simulink library "commchan2"  (Simulink 6.0)
settings: Solver=ode45  SolverMode=SingleTasking  StartTime=0.0  StopTime=10.0  RelTol=1e-3
undefined symbols (not defined in the file or in its folder): j, params
libraries: dspmlti3 x5, dspsigattribs x4, dspsrcs4 x3, commblksprivate x2, dspmtrx3 x2, dsparch4 x1, dspsigops x1, commchan2 x1
settings Model: RequirementInfo=9  CovMetricSettings=d  Creator=tdelve  LastModifiedBy=cvora  ExtModeAutoUpdateStatusClock=off  ProdHWDeviceType=Specified
settings DataIOCC: SignalLoggingName=logsOut
settings OptimizationCC: BooleanDataType=off
settings DebuggingCC: CheckExecutionContextPreStartOutputMsg=on  CheckExecutionContextRuntimeOutputMsg=on  SolverPrmCheckMsg=none
settings HardwareCC: ProdHWDeviceType=Specified
settings SFSimCC: SFSimApplyToAllLibs=on  SFSimBuildMode=Incremental

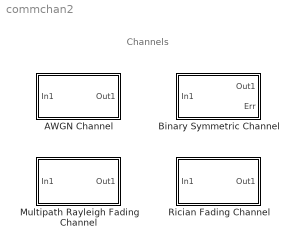
== system commchan2 ==
  note: Channels
  AWGN Channel : Subsystem  PropExecContextAcrossSSBoundary=on  mask(AWGN Channel){seed=67, noiseMode=Signal to noise ratio  (Eb/No), EbNodB=10, EsNodB=10, SNRdB=10, bitsPerSym=1, Ps=1, Tsym=1, variance=1}
      mask prompts: seed "Initial seed:"; noiseMode "Mode:"; EbNodB "Eb/No (dB):"; EsNodB "Es/No (dB):"; SNRdB "SNR (dB):"; bitsPerSym "Number of bits per symbol:"; Ps "Input signal power (watts):"; Tsym "Symbol period (s):"
      mask help:
      | Add white Gaussian noise to the input signal. The input and output signals can be real or complex. This block supports multichannel input and output signals as well as frame-based processing.
      |
      | When using either of the variance modes with complex inputs, the variance values are equally divided among the real and imaginary components of the input signal.
      mask init:
      | [mode,s]=commblkawgnchan2(gcb,'init');
      | if ~isempty(s.status) error(s.status); end
      mask Help: helpview(commbhelp)
      mask StyleString: edit,popup(Signal to noise ratio  (Eb/No)|Signal to noise ratio  (Es/No)|Signal to noise ratio  (SNR)|Variance from mask|Variance from port),edit,edit,edit,edit,edit,edit,edit
      mask CallbackString: |commblkawgnchan2(gcb,'Mode');|||||||
      mask Display:
      | plot(-10,-10,110, 110,[05 15 10 10 05 10 18 14 13 7.5 13 41 44 47 50 53 57
      | 59 100-[13 7.5 13 14 18 10 5 10 10 15 5]],[70 70 70 85 92 85 79 82 90 88.5
      | 90 90 87 93 87 93 87 90 90 88.5 90 82 79 85 92 85 70 70 70]);
      | disp('AWGN');
      | port_label('input',s.i1,s.i1s);
      | port_label('input',s.i2,s.i2s);
      | port_label('output',s.o1,s.o1s);
  Binary Symmetric Channel : Subsystem  PropExecContextAcrossSSBoundary=on  mask(Binary Symmetric Channel){P=0.05, s=71, E=on}
      mask prompts: P "Error probability:"; s "Initial seed:"; E "Output error vector"
      mask help:
      | Add binary errors to the input signal. The error probability can be a scalar or a vector with the same length as the input vector length.
      |
      | The optional second output is the error vector.
      mask init:
      | blk_icon = commblkbschan(P,s);
      mask Help: helpview(commbhelp)
      mask Display:
      | plot(0,0,100,100,[05 15 10 10 05 10 18 14 13 7.5 13 41 44 47 50 53 57 59 100-[13 7.5 13 14 18 10 5 10 10 15 5]],[70 70 70 85 92 85 79 82 90 88.5 90 90 87 93 87 93 87 90 90 88.5 90 82 79 85 92 85 70 70 70]);
      | disp('BSC')
      | port_label('output',blk_icon.portnum,blk_icon.portlabel);
  Multipath Rayleigh Fading Channel : Subsystem  PropExecContextAcrossSSBoundary=on  mask(Multipath Rayleigh Fading Channel){Fd=40, simTs=1e-6, delayVec=[0 2e-6], gainVecdB=[0 -3], normGain=on, Seed=73}
      mask prompts: Fd "Maximum Doppler shift (Hz):"; simTs "Sample time:"; delayVec "Delay vector (s):"; gainVecdB "Gain vector (dB):"; normGain "Normalize gain vector to 0 dB overall gain"; Seed "Initial seed:"
      mask help:
      | Multipath Rayleigh fading channel for complex baseband signals.
      |
      | Multiplies the input signal with samples of a Rayleigh distributed complex random process. The spectrum of the Rayleigh process is given by the Jakes PSD.
      |
      | The number of paths equals the length of either the 'Delay vector' or 'Gain vector' parameters.
      mask init:
      | commblkrayleighchan2(gcb);
      mask Help: helpview(commbhelp)
      mask Display:
      | plot(0,0,100,100,[05 15 10 10 05 10 18 14 13 7.5 13 41 44 47 50 53 57 59 100-[13 7.5 13 14 18 10 5 10 10 15 5]],[70 70 70 85 92 85 79 82 90 88.5 90 90 87 93 87 93 87 90 90 88.5 90 82 79 85 92 85 70 70 70]);
      | disp('Multipath\nRayleigh Fading')
  Rician Fading Channel : Subsystem  PropExecContextAcrossSSBoundary=on  mask(Rician Fading Channel){K=1, Fd=40, simTs=1e-6, delayVec=0, gainVecdB=0, Seed=79}
      mask prompts: K "K-factor:"; Fd "Maximum Doppler shift (Hz):"; simTs "Sample time:"; delayVec "Delay (s):"; gainVecdB "Gain (dB):"; Seed "Initial seed:"
      mask help:
      | Rician fading channel for complex baseband signals.
      |
      | Multiplies the input signal with samples of a Rician distributed complex random process. The K-factor parameter specifies the linear ratio of power in the direct path to the diffuse power.  The spectrum of the Rician process is given by the Jakes PSD.
      mask init:
      | commblkricianchan2(gcb);
      mask Help: helpview(commbhelp)
      mask Display:
      | plot(0,0,100,100,[05 15 10 10 05 10 18 14 13 7.5 13 41 44 47 50 53 57 59 100-[13 7.5 13 14 18 10 5 10 10 15 5]],[70 70 70 85 92 85 79 82 90 88.5 90 90 87 93 87 93 87 90 90 88.5 90 82 79 85 92 85 70 70 70]);
      | disp('Rician\nFading')

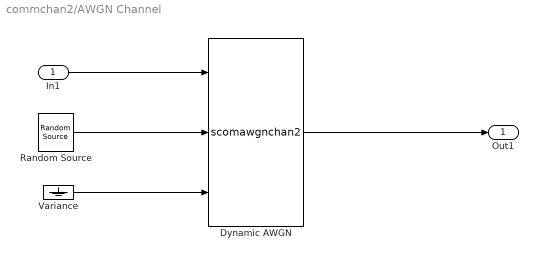
== system commchan2/AWGN Channel ==
  In1 : Inport  LatchInput=off
  Dynamic AWGN : S-Function  FunctionName=scomawgnchan2  Parameters=noiseMode, EbNodB, EsNodB, SNRdB, bitsPerSym, Ps, Tsym, variance
  Random Source : dspsrcs4/Random Source  SrcType=Gaussian  NormMethod=Ziggurat  CltLength=12  Min=0  Max=1  Mean=0  Var=1  RepMode=Specify seed  Seed=seed  Inherit=on  SampMode=Discrete  SampTime=1  SampFrame=1  DataType=Double  OutComplex=Real
  Variance : Ground
  Out1 : Outport
  wires:
  Random Source/1 -> Dynamic AWGN/2
  In1/1 -> Dynamic AWGN/1
  Dynamic AWGN/1 -> Out1/1
  Variance/1 -> Dynamic AWGN/3

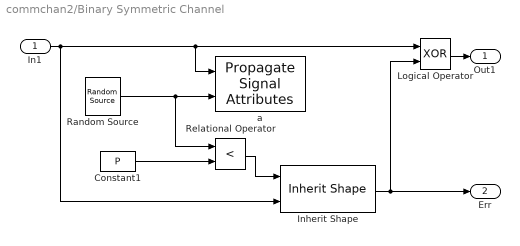
== system commchan2/Binary Symmetric Channel ==
  In1 : Inport  LatchInput=off
  Constant1 : Constant  Value=P
  Inherit Shape : commblksprivate/Inherit Shape
  Logical Operator : Logic  Operator=XOR  OutDataTypeMode=Specify via dialog  LogicDataType=float('double')
  Random Source : dspsrcs4/Random Source  SrcType=Uniform  NormMethod=Ziggurat  CltLength=12  Min=0  Max=1  Mean=0  Var=1  RepMode=Specify seed  Seed=s  Inherit=on  SampMode=Discrete  SampTime=1  SampFrame=1  DataType=Double  OutComplex=Real
  Relational Operator : RelationalOperator  Operator=<  LogicOutDataTypeMode=Specify via dialog  LogicDataType=float('double')  InputSameDT=on
  a : commblksprivate/Propagate Signal Attributes
  Out1 : Outport
  Err : Outport  Port=2
  wires:
  Relational Operator/1 -> Inherit Shape/1
  Inherit Shape/1 -> Logical Operator/2, Err/1
  Logical Operator/1 -> Out1/1
  In1/1 -> Inherit Shape/2, Logical Operator/1, a/1
  Constant1/1 -> Relational Operator/2
  Random Source/1 -> Relational Operator/1, a/2

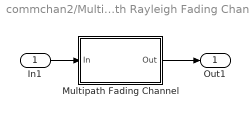
== system commchan2/Multipath Rayleigh Fading Channel ==
  In1 : Inport  LatchInput=off
  Multipath Fading Channel : Subsystem  PropExecContextAcrossSSBoundary=on  mask(Multipath Fading Channel){Fd=Fd, LOSFd=0, K=0, simTs=simTs, delayVec=delayVec, gainVecdB=gainVecdB, normGain=on, Seed=Seed}
      mask prompts: Fd "Doppler frequency (Hz):"; LOSFd "Line-of-sight Doppler frequency (Hz):"; K "K-factor:"; simTs "Sample time (sec):"; delayVec "Delay vector (sec):"; gainVecdB "Gain vector (dB):"; normGain "Normalize gain vector to 0 dB overall gain"; Seed "Initial seed:"
      mask help:
      | Multipath fading channel for complex baseband signals.
      |
      | Multiplies the input signal with samples of a complex random process. The spectrum of the random process is given by the Jakes PSD, where the Doppler frequency parameter determines the maximum Doppler frequency. The K-factor parameter specifies the linear ratio of power in the direct path to the diffuse power.
      |
      | The number of paths equals the length of either the 'Delay vector' or 'Gain vector' parameters.
      mask init:
      | [ecode,emsg,params] = commblkfadingchan2(gcb,Fd,LOSFd,K,simTs,delayVec,gainVecdB,normGain,Seed);
      | if(ecode==1)
      |     error(emsg);
      | elseif(ecode==2)
      |     warning(emsg);
      | end;
      mask Display:
      | plot(0,0,100,100,[05 15 10 10 05 10 18 14 13 7.5 13 41 44 47 50 53 57 59 100-[13 7.5 13 14 18 10 5 10 10 15 5]],[70 70 70 85 92 85 79 82 90 88.5 90 90 87 93 87 93 87 90 90 88.5 90 82 79 85 92 85 70 70 70]);
      | disp('Multipath\nFading')
  Out1 : Outport
  wires:
  In1/1 -> Multipath Fading Channel/1(In)
  Multipath Fading Channel/1(Out) -> Out1/1

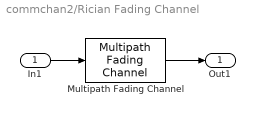
== system commchan2/Rician Fading Channel ==
  In1 : Inport  LatchInput=off
  Multipath Fading Channel : commchan2/Multipath Rayleigh Fading Channel/Multipath Fading Channel  Fd=Fd  LOSFd=0  K=K  simTs=simTs  delayVec=delayVec  gainVecdB=gainVecdB  normGain=off  Seed=Seed
  Out1 : Outport
  wires:
  In1/1 -> Multipath Fading Channel/1
  Multipath Fading Channel/1 -> Out1/1

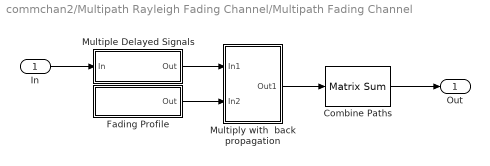
== system commchan2/Multipath Rayleigh Fading Channel/Multipath Fading Channel ==
  In : Inport  LatchInput=off
  Combine Paths : dspmtrx3/Matrix Sum  DialogController=dspDDGCreate  DialogControllerArgs=DataTag0  Dim=Rows  roundingMode=Floor  overflowMode=off
  Fading Profile : Subsystem  PropExecContextAcrossSSBoundary=on
      mask Display: disp('Fading\nProfile')
  Multiple Delayed Signals : Subsystem  PropExecContextAcrossSSBoundary=on  mask(Multiple Delayed Signals){delayVector=params.sampleDelayVec, Ts=simTs}
      mask prompts: delayVector "Path delay vector:"; Ts "Sample time (sec):"
      mask init:
      | nPaths = length(delayVector);
      | maxDelay = ceil(max(delayVector))+1;
      mask Display: disp('Multiple\ndelayed signals');
  Multiply with  back propagation : Subsystem  PropExecContextAcrossSSBoundary=on  mask(Multiply with back propagation){propTarget=Input 2, Ts=simTs, numChan=params.nPaths}
      mask prompts: propTarget "Propagation target:"; Ts "Sample time:"; numChan "Number of channels:"
      mask help:
      | Perform multiplication of the two input signals.
      |
      | The width and complexity of the output and the port not targeted for propagation must be identical. The width and complexity of the port targeted for propagation is set to that of the other input.
      |
      | The block sample time is the product of the number of samples per frame and the sample time parameter.
      mask StyleString: popup(Input 1|Input 2),edit,edit
      mask Display: disp('Multiply\nwith prop');
  Out : Outport
  wires:
  Multiple Delayed Signals/1(Out) -> Multiply with  back propagation/1(In1)
  Fading Profile/1(Out) -> Multiply with  back propagation/2(In2)
  In/1 -> Multiple Delayed Signals/1(In)
  Multiply with  back propagation/1(Out1) -> Combine Paths/1
  Combine Paths/1 -> Out/1

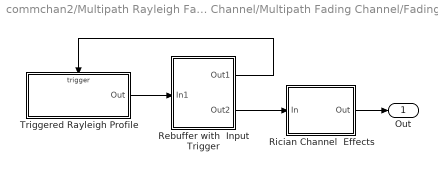
== system commchan2/Multipath Rayleigh Fading Channel/Multipath Fading Channel/Fading Profile ==
  Rebuffer with  Input Trigger : Subsystem  PropExecContextAcrossSSBoundary=on  mask(Rebuffer with Input Trigger){startSample=params.startDelay, numChan=params.nPaths, inputWidthMode=Based on output width, inputWidth=params.intFactor, inputWidthMin=params.intFactor, inputWidthStep=params.intFactor}
      mask prompts: startSample "Start delay:"; numChan "Number of channels:"; inputWidthMode "Input width mode:"; inputWidth "Input width (per channel):"; inputWidthMin "Minimum input width (per channel):"; inputWidthStep "Input width step size (per channel):"
      mask help: This block inherits the input and output port widths and complexity and the output sample time. The input must be from a function call subsystem. The block generates a function call trigger on port 1 when ever data is required. and outputs the buffered input data on port 2.
      mask init:
      | s = commblktriggeredbuffer(gcb,'init',{});
      mask StyleString: edit,edit,popup(Inherit|Specify|Based on output width),edit,edit,edit
      mask CallbackString: ||commblktriggeredbuffer(gcb,'InputWidthMode');|||
      mask Display:
      | disp('Rebuffer\nwith trigger');
      | port_label('input',s.i1,s.i1s);
      | port_label('output',s.o1,s.o1s);
      | port_label('output',s.o2,s.o2s);
  Rician Channel  Effects : Subsystem  PropExecContextAcrossSSBoundary=on  mask(Ricean Channel Effects){Doppler=params.LOSFd, K=params.K, opPower=params.gainVecLin, Ts=simTs, numChan=params.nPaths}
      mask prompts: Doppler "Line-of-sight Doppler frequency (Hz):"; K "K-factor"; opPower "Required output power (Watts):"; Ts "Sample time (s):"; numChan "Number of channels:"
      mask help: Add a complex phasor to the unity variance complex input to produce Rician channel effects. The Doppler frequency parameter determines frequency of the complex phasor.
      mask Display: disp('Rician\nChannel')
  Triggered Rayleigh Profile : Subsystem  TreatAsAtomicUnit=on  PropExecContextAcrossSSBoundary=on
  Out : Outport
  wires:
  Triggered Rayleigh Profile/1(Out) -> Rebuffer with  Input Trigger/1(In1)
  Rebuffer with  Input Trigger/1(Out1) -> Triggered Rayleigh Profile/Trigger
  Rician Channel  Effects/1(Out) -> Out/1
  Rebuffer with  Input Trigger/2(Out2) -> Rician Channel  Effects/1(In)

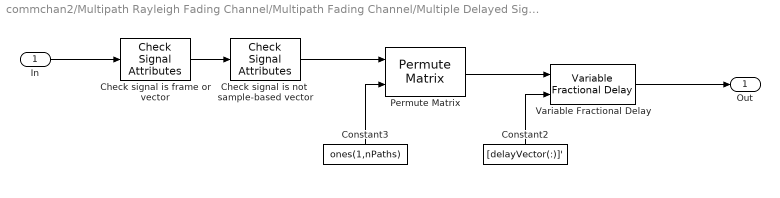
== system commchan2/Multipath Rayleigh Fading Channel/Multipath Fading Channel/Multiple Delayed Signals ==
  In : Inport  LatchInput=off
  Check signal is frame or vector : dspsigattribs/Check Signal Attributes  SigAttribCheckMethod=Does not match attributes exactly  Complexity=Ignore  Frame=Ignore  DimsCheckMethod=Is...  Dimensions=Column vector (2-D) or scalar  DatatypeCheckMethod=Ignore  DatatypeGeneral=Boolean  DtypeFloatSpecific=Any floating-point  DtypeFixedSpecific=Any fixed-point  DtypeIntSpecific=Any integer  SampleMode=Ignore
  Check signal is not  sample-based vector : dspsigattribs/Check Signal Attributes  SigAttribCheckMethod=Matches attributes exactly  Complexity=Ignore  Frame=Sample-based  DimsCheckMethod=Is not...  Dimensions=Scalar (1-D or 2-D)  DatatypeCheckMethod=Ignore  DatatypeGeneral=Boolean  DtypeFloatSpecific=Any floating-point  DtypeFixedSpecific=Any fixed-point  DtypeIntSpecific=Any integer  SampleMode=Ignore
  Constant2 : Constant  Orientation=up  Value=[delayVector(:)]'  VectorParams1D=off
  Constant3 : Constant  Orientation=up  Value=ones(1,nPaths)  VectorParams1D=off
  Permute Matrix : dspmtrx3/Permute Matrix  mode=Columns  ZeroOneIdxMode=One-based  errmode=Clip Index  checkDims=off
  Variable Fractional Delay : dspsigops/Variable Fractional Delay  mode=FIR Interpolation  dmax=maxDelay  L=6  R=10  alpha=1  ic=0
  Out : Outport
  wires:
  Variable Fractional Delay/1 -> Out/1
  Check signal is frame or vector/1 -> Check signal is not  sample-based vector/1
  Permute Matrix/1 -> Variable Fractional Delay/1
  Constant3/1 -> Permute Matrix/2
  Constant2/1 -> Variable Fractional Delay/2
  In/1 -> Check signal is frame or vector/1
  Check signal is not  sample-based vector/1 -> Permute Matrix/1

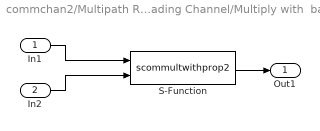
== system commchan2/Multipath Rayleigh Fading Channel/Multipath Fading Channel/Multiply with  back propagation ==
  In1 : Inport  LatchInput=off
  In2 : Inport  Port=2  LatchInput=off
  S-Function : S-Function  FunctionName=scommultwithprop2  Parameters=propTarget, Ts, numChan
  Out1 : Outport
  wires:
  S-Function/1 -> Out1/1
  In1/1 -> S-Function/1
  In2/1 -> S-Function/2

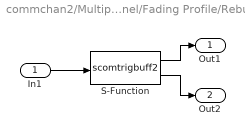
== system commchan2/Multipath Rayleigh Fading Channel/Multipath Fading Channel/Fading Profile/Rebuffer with  Input Trigger ==
  In1 : Inport  LatchInput=off
  S-Function : S-Function  FunctionName=scomtrigbuff2  Parameters=startSample, numChan, inputWidthMode, inputWidth, inputWidthMin, inputWidthStep
  Out1 : Outport
  Out2 : Outport  Port=2
  wires:
  In1/1 -> S-Function/1
  S-Function/2 -> Out2/1
  S-Function/1 -> Out1/1

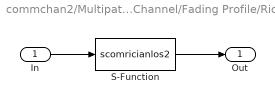
== system commchan2/Multipath Rayleigh Fading Channel/Multipath Fading Channel/Fading Profile/Rician Channel  Effects ==
  In : Inport  LatchInput=off
  S-Function : S-Function  FunctionName=scomricianlos2  Parameters=Doppler,K,opPower,Ts,numChan
  Out : Outport
  wires:
  S-Function/1 -> Out/1
  In/1 -> S-Function/1

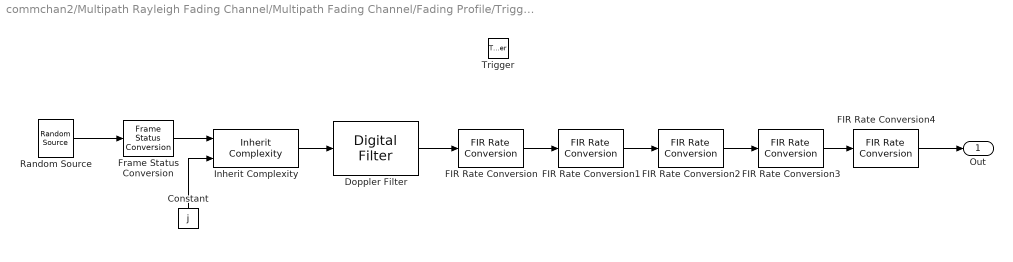
== system commchan2/Multipath Rayleigh Fading Channel/Multipath Fading Channel/Fading Profile/Triggered Rayleigh Profile ==
  Trigger : TriggerPort  TriggerType=function-call
  Constant : Constant  Orientation=up  Value=j
  Doppler Filter : dsparch4/Digital Filter  TypePopup=IIR (poles & zeros)  IIRFiltStruct=Biquad direct form II transposed (SOS)  AllPoleFiltStruct=Direct form  FIRFiltStruct=Direct form  CoeffSource=Specify via dialog  NumCoeffs=[1 2]  DenCoeffs=[1 0.1]  BiQuadCoeffs=params.dopplerSos  LatticeCoeffs=[0.2 0.4]  denIgnore=on  FiltPerSampPopup=One filter per frame  IC=0  ICnum=0  ICden=0
  FIR Rate Conversion : dspmlti3/FIR Rate Conversion  L=params.interp1  h=params.rc1Num  M=params.decim1
  FIR Rate Conversion1 : dspmlti3/FIR Rate Conversion  L=params.interp2  h=params.rc2Num  M=params.decim2
  FIR Rate Conversion2 : dspmlti3/FIR Rate Conversion  L=params.interp3  h=params.rc3Num  M=params.decim3
  FIR Rate Conversion3 : dspmlti3/FIR Rate Conversion  L=params.interp4  h=params.rc4Num  M=params.decim4
  FIR Rate Conversion4 : dspmlti3/FIR Rate Conversion  L=params.interp5  h=params.rc5Num  M=params.decim5
  Frame Status Conversion : dspsigattribs/Frame Status Conversion  growRefPort=off  outframe=Frame-based
  Inherit Complexity : dspsigattribs/Inherit Complexity
  Random Source : dspsrcs4/Random Source  SrcType=Gaussian  NormMethod=Ziggurat  CltLength=12  Min=0  Max=1  Mean=0  Var=1  RepMode=Specify seed  Seed=params.Seed  Inherit=on  SampMode=Discrete  SampTime=1  SampFrame=1  DataType=Double  OutComplex=Real
  Out : Outport
  wires:
  FIR Rate Conversion3/1 -> FIR Rate Conversion4/1
  FIR Rate Conversion2/1 -> FIR Rate Conversion3/1
  Frame Status Conversion/1 -> Inherit Complexity/1
  Random Source/1 -> Frame Status Conversion/1
  Constant/1 -> Inherit Complexity/2
  Inherit Complexity/1 -> Doppler Filter/1
  FIR Rate Conversion/1 -> FIR Rate Conversion1/1
  Doppler Filter/1 -> FIR Rate Conversion/1
  FIR Rate Conversion1/1 -> FIR Rate Conversion2/1
  FIR Rate Conversion4/1 -> Out/1
